simulink model "InjCtl"  (R2018a)
settings: configuration reference "cs_ert" (kept outside this file)
settings Model: DataDictionary=InjCtl.sldd  Creator=zhoutinglin  LastModifiedBy=zhoutinglin

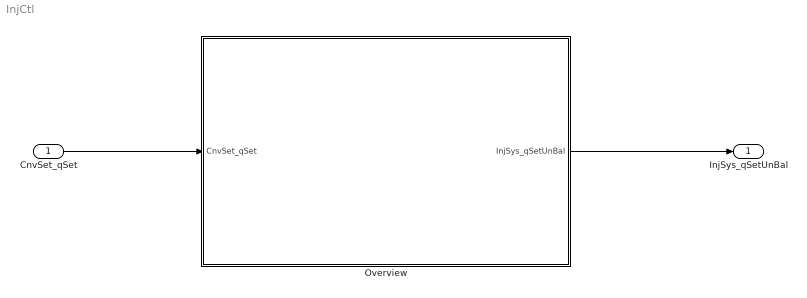
== system InjCtl ==
  CnvSet_qSet : Inport
  Overview : Subsystem
  InjSys_qSetUnBal : Outport
  wires:
  CnvSet_qSet/1 -> Overview/1(CnvSet_qSet)
  Overview/1(InjSys_qSetUnBal) -> InjSys_qSetUnBal/1

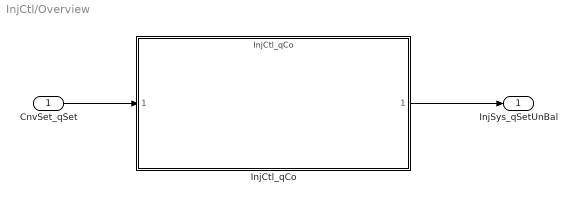
== system InjCtl/Overview ==
  CnvSet_qSet : Inport
  InjCtl_qCo : ModelReference  ModelNameDialog=InjCtl_qCo  SimulationMode=Normal  ModelReferenceVersion=1.58
  InjSys_qSetUnBal : Outport
  wires:
  InjCtl_qCo/1 -> InjSys_qSetUnBal/1
  CnvSet_qSet/1 -> InjCtl_qCo/1
